simulink model "generic"  (R2021a)
settings: Solver=ode8  StartTime=0.0  StopTime=inf  FixedStep=0.001  RelTol=1e-3  EnableMultiTasking=on
StartFcn:
  | addpath('C:\Stud\Mgr_work\casadi-windows-matlabR2016a-v3.5.5')
  | import casadi.*
libraries: CarMaker4SL x35, simulink x1
(part 3 of 3)

== system generic/CarMaker/VehicleControl/CreateBus VhclCtrl/Environmental Envelope Protection/MPC/for ruts/Subsystem3 ==
  In1 : Inport
  Bus Selector{1..10} (10 alike) : BusSelector  OutputSignals=x,y,z
  Mux : Mux  Inputs=10
  Mux1 : Mux  Inputs=10
  Selector1 : Selector  InputPortWidth=200  IndexOptions=Index vector (dialog)  Indices=1  OutputSizes=1
  Selector10 : Selector  InputPortWidth=200  IndexOptions=Index vector (dialog)  Indices=10  OutputSizes=1
  Selector2 : Selector  InputPortWidth=200  IndexOptions=Index vector (dialog)  Indices=2  OutputSizes=1
  Selector3 : Selector  InputPortWidth=200  IndexOptions=Index vector (dialog)  Indices=3  OutputSizes=1
  Selector4 : Selector  InputPortWidth=200  IndexOptions=Index vector (dialog)  Indices=4  OutputSizes=1
  Selector5 : Selector  InputPortWidth=200  IndexOptions=Index vector (dialog)  Indices=5  OutputSizes=1
  Selector6 : Selector  InputPortWidth=200  IndexOptions=Index vector (dialog)  Indices=6  OutputSizes=1
  Selector7 : Selector  InputPortWidth=200  IndexOptions=Index vector (dialog)  Indices=7  OutputSizes=1
  Selector8 : Selector  InputPortWidth=200  IndexOptions=Index vector (dialog)  Indices=8  OutputSizes=1
  Selector9 : Selector  InputPortWidth=200  IndexOptions=Index vector (dialog)  Indices=9  OutputSizes=1
  x : Outport
  y : Outport  Port=2
  wires:
  Bus Selector1/1 -> Mux/1  "<x>"
  Bus Selector2/2 -> Mux1/2  "<y>"
  In1/1 -> Selector2/1, Selector10/1, Selector9/1, Selector8/1, Selector7/1, Selector6/1, Selector5/1, Selector4/1, Selector3/1, Selector1/1
  Bus Selector2/1 -> Mux/2  "<x>"
  Selector2/1 -> Bus Selector2/1
  Selector1/1 -> Bus Selector1/1
  Bus Selector1/2 -> Mux1/1  "<y>"
  Bus Selector3/1 -> Mux/3  "<x>"
  Bus Selector3/2 -> Mux1/3  "<y>"
  Selector3/1 -> Bus Selector3/1
  Bus Selector4/1 -> Mux/4  "<x>"
  Bus Selector4/2 -> Mux1/4  "<y>"
  Selector4/1 -> Bus Selector4/1
  Bus Selector5/1 -> Mux/5  "<x>"
  Bus Selector5/2 -> Mux1/5  "<y>"
  Selector5/1 -> Bus Selector5/1
  Bus Selector6/1 -> Mux/6  "<x>"
  Bus Selector6/2 -> Mux1/6  "<y>"
  Selector6/1 -> Bus Selector6/1
  Bus Selector7/1 -> Mux/7  "<x>"
  Bus Selector7/2 -> Mux1/7  "<y>"
  Selector7/1 -> Bus Selector7/1
  Bus Selector8/1 -> Mux/8  "<x>"
  Bus Selector8/2 -> Mux1/8  "<y>"
  Selector8/1 -> Bus Selector8/1
  Bus Selector9/1 -> Mux/9  "<x>"
  Bus Selector9/2 -> Mux1/9  "<y>"
  Selector9/1 -> Bus Selector9/1
  Bus Selector10/1 -> Mux/10  "<x>"
  Bus Selector10/2 -> Mux1/10  "<y>"
  Selector10/1 -> Bus Selector10/1
  Mux1/1 -> y/1
  Mux/1 -> x/1

== system generic/CarMaker/VehicleControl/CreateBus VhclCtrl/Environmental Envelope Protection/MPC/for ruts/Subsystem4 ==
  In1 : Inport
  Bus Selector{1..10} (10 alike) : BusSelector  OutputSignals=x,y,z
  Mux : Mux  Inputs=10
  Mux1 : Mux  Inputs=10
  Selector1 : Selector  InputPortWidth=200  IndexOptions=Index vector (dialog)  Indices=1  OutputSizes=1
  Selector10 : Selector  InputPortWidth=200  IndexOptions=Index vector (dialog)  Indices=10  OutputSizes=1
  Selector2 : Selector  InputPortWidth=200  IndexOptions=Index vector (dialog)  Indices=2  OutputSizes=1
  Selector3 : Selector  InputPortWidth=200  IndexOptions=Index vector (dialog)  Indices=3  OutputSizes=1
  Selector4 : Selector  InputPortWidth=200  IndexOptions=Index vector (dialog)  Indices=4  OutputSizes=1
  Selector5 : Selector  InputPortWidth=200  IndexOptions=Index vector (dialog)  Indices=5  OutputSizes=1
  Selector6 : Selector  InputPortWidth=200  IndexOptions=Index vector (dialog)  Indices=6  OutputSizes=1
  Selector7 : Selector  InputPortWidth=200  IndexOptions=Index vector (dialog)  Indices=7  OutputSizes=1
  Selector8 : Selector  InputPortWidth=200  IndexOptions=Index vector (dialog)  Indices=8  OutputSizes=1
  Selector9 : Selector  InputPortWidth=200  IndexOptions=Index vector (dialog)  Indices=9  OutputSizes=1
  x : Outport
  y : Outport  Port=2
  wires:
  Bus Selector1/1 -> Mux/1  "<x>"
  Bus Selector2/2 -> Mux1/2  "<y>"
  In1/1 -> Selector2/1, Selector10/1, Selector9/1, Selector8/1, Selector7/1, Selector6/1, Selector5/1, Selector4/1, Selector3/1, Selector1/1
  Bus Selector2/1 -> Mux/2  "<x>"
  Selector2/1 -> Bus Selector2/1
  Selector1/1 -> Bus Selector1/1
  Bus Selector1/2 -> Mux1/1  "<y>"
  Bus Selector3/1 -> Mux/3  "<x>"
  Bus Selector3/2 -> Mux1/3  "<y>"
  Selector3/1 -> Bus Selector3/1
  Bus Selector4/1 -> Mux/4  "<x>"
  Bus Selector4/2 -> Mux1/4  "<y>"
  Selector4/1 -> Bus Selector4/1
  Bus Selector5/1 -> Mux/5  "<x>"
  Bus Selector5/2 -> Mux1/5  "<y>"
  Selector5/1 -> Bus Selector5/1
  Bus Selector6/1 -> Mux/6  "<x>"
  Bus Selector6/2 -> Mux1/6  "<y>"
  Selector6/1 -> Bus Selector6/1
  Bus Selector7/1 -> Mux/7  "<x>"
  Bus Selector7/2 -> Mux1/7  "<y>"
  Selector7/1 -> Bus Selector7/1
  Bus Selector8/1 -> Mux/8  "<x>"
  Bus Selector8/2 -> Mux1/8  "<y>"
  Selector8/1 -> Bus Selector8/1
  Bus Selector9/1 -> Mux/9  "<x>"
  Bus Selector9/2 -> Mux1/9  "<y>"
  Selector9/1 -> Bus Selector9/1
  Bus Selector10/1 -> Mux/10  "<x>"
  Bus Selector10/2 -> Mux1/10  "<y>"
  Selector10/1 -> Bus Selector10/1
  Mux1/1 -> y/1
  Mux/1 -> x/1

== system generic/CarMaker/VehicleControl/CreateBus VhclCtrl/Environmental Envelope Protection/MPC/for ruts/Subsystem5 ==
  In1 : Inport
  Bus Selector{1..10} (10 alike) : BusSelector  OutputSignals=x,y,z
  Mux : Mux  Inputs=10
  Mux1 : Mux  Inputs=10
  Selector1 : Selector  InputPortWidth=200  IndexOptions=Index vector (dialog)  Indices=1  OutputSizes=1
  Selector10 : Selector  InputPortWidth=200  IndexOptions=Index vector (dialog)  Indices=10  OutputSizes=1
  Selector2 : Selector  InputPortWidth=200  IndexOptions=Index vector (dialog)  Indices=2  OutputSizes=1
  Selector3 : Selector  InputPortWidth=200  IndexOptions=Index vector (dialog)  Indices=3  OutputSizes=1
  Selector4 : Selector  InputPortWidth=200  IndexOptions=Index vector (dialog)  Indices=4  OutputSizes=1
  Selector5 : Selector  InputPortWidth=200  IndexOptions=Index vector (dialog)  Indices=5  OutputSizes=1
  Selector6 : Selector  InputPortWidth=200  IndexOptions=Index vector (dialog)  Indices=6  OutputSizes=1
  Selector7 : Selector  InputPortWidth=200  IndexOptions=Index vector (dialog)  Indices=7  OutputSizes=1
  Selector8 : Selector  InputPortWidth=200  IndexOptions=Index vector (dialog)  Indices=8  OutputSizes=1
  Selector9 : Selector  InputPortWidth=200  IndexOptions=Index vector (dialog)  Indices=9  OutputSizes=1
  x : Outport
  y : Outport  Port=2
  wires:
  Bus Selector1/1 -> Mux/1  "<x>"
  Bus Selector2/2 -> Mux1/2  "<y>"
  In1/1 -> Selector2/1, Selector10/1, Selector9/1, Selector8/1, Selector7/1, Selector6/1, Selector5/1, Selector4/1, Selector3/1, Selector1/1
  Bus Selector2/1 -> Mux/2  "<x>"
  Selector2/1 -> Bus Selector2/1
  Selector1/1 -> Bus Selector1/1
  Bus Selector1/2 -> Mux1/1  "<y>"
  Bus Selector3/1 -> Mux/3  "<x>"
  Bus Selector3/2 -> Mux1/3  "<y>"
  Selector3/1 -> Bus Selector3/1
  Bus Selector4/1 -> Mux/4  "<x>"
  Bus Selector4/2 -> Mux1/4  "<y>"
  Selector4/1 -> Bus Selector4/1
  Bus Selector5/1 -> Mux/5  "<x>"
  Bus Selector5/2 -> Mux1/5  "<y>"
  Selector5/1 -> Bus Selector5/1
  Bus Selector6/1 -> Mux/6  "<x>"
  Bus Selector6/2 -> Mux1/6  "<y>"
  Selector6/1 -> Bus Selector6/1
  Bus Selector7/1 -> Mux/7  "<x>"
  Bus Selector7/2 -> Mux1/7  "<y>"
  Selector7/1 -> Bus Selector7/1
  Bus Selector8/1 -> Mux/8  "<x>"
  Bus Selector8/2 -> Mux1/8  "<y>"
  Selector8/1 -> Bus Selector8/1
  Bus Selector9/1 -> Mux/9  "<x>"
  Bus Selector9/2 -> Mux1/9  "<y>"
  Selector9/1 -> Bus Selector9/1
  Bus Selector10/1 -> Mux/10  "<x>"
  Bus Selector10/2 -> Mux1/10  "<y>"
  Selector10/1 -> Bus Selector10/1
  Mux1/1 -> y/1
  Mux/1 -> x/1

== system generic/CarMaker/VehicleControl/CreateBus VhclCtrl/Environmental Envelope Protection/MPC/for ruts/Subsystem6 ==
  In1 : Inport
  Bus Selector{1..10} (10 alike) : BusSelector  OutputSignals=x,y,z
  Mux : Mux  Inputs=10
  Mux1 : Mux  Inputs=10
  Selector1 : Selector  InputPortWidth=200  IndexOptions=Index vector (dialog)  Indices=1  OutputSizes=1
  Selector10 : Selector  InputPortWidth=200  IndexOptions=Index vector (dialog)  Indices=10  OutputSizes=1
  Selector2 : Selector  InputPortWidth=200  IndexOptions=Index vector (dialog)  Indices=2  OutputSizes=1
  Selector3 : Selector  InputPortWidth=200  IndexOptions=Index vector (dialog)  Indices=3  OutputSizes=1
  Selector4 : Selector  InputPortWidth=200  IndexOptions=Index vector (dialog)  Indices=4  OutputSizes=1
  Selector5 : Selector  InputPortWidth=200  IndexOptions=Index vector (dialog)  Indices=5  OutputSizes=1
  Selector6 : Selector  InputPortWidth=200  IndexOptions=Index vector (dialog)  Indices=6  OutputSizes=1
  Selector7 : Selector  InputPortWidth=200  IndexOptions=Index vector (dialog)  Indices=7  OutputSizes=1
  Selector8 : Selector  InputPortWidth=200  IndexOptions=Index vector (dialog)  Indices=8  OutputSizes=1
  Selector9 : Selector  InputPortWidth=200  IndexOptions=Index vector (dialog)  Indices=9  OutputSizes=1
  x : Outport
  y : Outport  Port=2
  wires:
  Bus Selector1/1 -> Mux/1  "<x>"
  Bus Selector2/2 -> Mux1/2  "<y>"
  In1/1 -> Selector2/1, Selector10/1, Selector9/1, Selector8/1, Selector7/1, Selector6/1, Selector5/1, Selector4/1, Selector3/1, Selector1/1
  Bus Selector2/1 -> Mux/2  "<x>"
  Selector2/1 -> Bus Selector2/1
  Selector1/1 -> Bus Selector1/1
  Bus Selector1/2 -> Mux1/1  "<y>"
  Bus Selector3/1 -> Mux/3  "<x>"
  Bus Selector3/2 -> Mux1/3  "<y>"
  Selector3/1 -> Bus Selector3/1
  Bus Selector4/1 -> Mux/4  "<x>"
  Bus Selector4/2 -> Mux1/4  "<y>"
  Selector4/1 -> Bus Selector4/1
  Bus Selector5/1 -> Mux/5  "<x>"
  Bus Selector5/2 -> Mux1/5  "<y>"
  Selector5/1 -> Bus Selector5/1
  Bus Selector6/1 -> Mux/6  "<x>"
  Bus Selector6/2 -> Mux1/6  "<y>"
  Selector6/1 -> Bus Selector6/1
  Bus Selector7/1 -> Mux/7  "<x>"
  Bus Selector7/2 -> Mux1/7  "<y>"
  Selector7/1 -> Bus Selector7/1
  Bus Selector8/1 -> Mux/8  "<x>"
  Bus Selector8/2 -> Mux1/8  "<y>"
  Selector8/1 -> Bus Selector8/1
  Bus Selector9/1 -> Mux/9  "<x>"
  Bus Selector9/2 -> Mux1/9  "<y>"
  Selector9/1 -> Bus Selector9/1
  Bus Selector10/1 -> Mux/10  "<x>"
  Bus Selector10/2 -> Mux1/10  "<y>"
  Selector10/1 -> Bus Selector10/1
  Mux1/1 -> y/1
  Mux/1 -> x/1

== system generic/CarMaker/VehicleControl/CreateBus VhclCtrl/Environmental Envelope Protection/MPC/for ruts/Subsystem7 ==
  In1 : Inport
  Bus Selector{1..10} (10 alike) : BusSelector  OutputSignals=x,y,z
  Mux : Mux  Inputs=10
  Mux1 : Mux  Inputs=10
  Selector1 : Selector  InputPortWidth=200  IndexOptions=Index vector (dialog)  Indices=1  OutputSizes=1
  Selector10 : Selector  InputPortWidth=200  IndexOptions=Index vector (dialog)  Indices=10  OutputSizes=1
  Selector2 : Selector  InputPortWidth=200  IndexOptions=Index vector (dialog)  Indices=2  OutputSizes=1
  Selector3 : Selector  InputPortWidth=200  IndexOptions=Index vector (dialog)  Indices=3  OutputSizes=1
  Selector4 : Selector  InputPortWidth=200  IndexOptions=Index vector (dialog)  Indices=4  OutputSizes=1
  Selector5 : Selector  InputPortWidth=200  IndexOptions=Index vector (dialog)  Indices=5  OutputSizes=1
  Selector6 : Selector  InputPortWidth=200  IndexOptions=Index vector (dialog)  Indices=6  OutputSizes=1
  Selector7 : Selector  InputPortWidth=200  IndexOptions=Index vector (dialog)  Indices=7  OutputSizes=1
  Selector8 : Selector  InputPortWidth=200  IndexOptions=Index vector (dialog)  Indices=8  OutputSizes=1
  Selector9 : Selector  InputPortWidth=200  IndexOptions=Index vector (dialog)  Indices=9  OutputSizes=1
  x : Outport
  y : Outport  Port=2
  wires:
  Bus Selector1/1 -> Mux/1  "<x>"
  Bus Selector2/2 -> Mux1/2  "<y>"
  In1/1 -> Selector2/1, Selector10/1, Selector9/1, Selector8/1, Selector7/1, Selector6/1, Selector5/1, Selector4/1, Selector3/1, Selector1/1
  Bus Selector2/1 -> Mux/2  "<x>"
  Selector2/1 -> Bus Selector2/1
  Selector1/1 -> Bus Selector1/1
  Bus Selector1/2 -> Mux1/1  "<y>"
  Bus Selector3/1 -> Mux/3  "<x>"
  Bus Selector3/2 -> Mux1/3  "<y>"
  Selector3/1 -> Bus Selector3/1
  Bus Selector4/1 -> Mux/4  "<x>"
  Bus Selector4/2 -> Mux1/4  "<y>"
  Selector4/1 -> Bus Selector4/1
  Bus Selector5/1 -> Mux/5  "<x>"
  Bus Selector5/2 -> Mux1/5  "<y>"
  Selector5/1 -> Bus Selector5/1
  Bus Selector6/1 -> Mux/6  "<x>"
  Bus Selector6/2 -> Mux1/6  "<y>"
  Selector6/1 -> Bus Selector6/1
  Bus Selector7/1 -> Mux/7  "<x>"
  Bus Selector7/2 -> Mux1/7  "<y>"
  Selector7/1 -> Bus Selector7/1
  Bus Selector8/1 -> Mux/8  "<x>"
  Bus Selector8/2 -> Mux1/8  "<y>"
  Selector8/1 -> Bus Selector8/1
  Bus Selector9/1 -> Mux/9  "<x>"
  Bus Selector9/2 -> Mux1/9  "<y>"
  Selector9/1 -> Bus Selector9/1
  Bus Selector10/1 -> Mux/10  "<x>"
  Bus Selector10/2 -> Mux1/10  "<y>"
  Selector10/1 -> Bus Selector10/1
  Mux1/1 -> y/1
  Mux/1 -> x/1

== system generic/CarMaker/VehicleControl/CreateBus VhclCtrl/Environmental Envelope Protection/MPC/for ruts/Subsystem8 ==
  In1 : Inport
  Bus Selector{1..10} (10 alike) : BusSelector  OutputSignals=x,y,z
  Mux : Mux  Inputs=10
  Mux1 : Mux  Inputs=10
  Selector1 : Selector  InputPortWidth=200  IndexOptions=Index vector (dialog)  Indices=1  OutputSizes=1
  Selector10 : Selector  InputPortWidth=200  IndexOptions=Index vector (dialog)  Indices=10  OutputSizes=1
  Selector2 : Selector  InputPortWidth=200  IndexOptions=Index vector (dialog)  Indices=2  OutputSizes=1
  Selector3 : Selector  InputPortWidth=200  IndexOptions=Index vector (dialog)  Indices=3  OutputSizes=1
  Selector4 : Selector  InputPortWidth=200  IndexOptions=Index vector (dialog)  Indices=4  OutputSizes=1
  Selector5 : Selector  InputPortWidth=200  IndexOptions=Index vector (dialog)  Indices=5  OutputSizes=1
  Selector6 : Selector  InputPortWidth=200  IndexOptions=Index vector (dialog)  Indices=6  OutputSizes=1
  Selector7 : Selector  InputPortWidth=200  IndexOptions=Index vector (dialog)  Indices=7  OutputSizes=1
  Selector8 : Selector  InputPortWidth=200  IndexOptions=Index vector (dialog)  Indices=8  OutputSizes=1
  Selector9 : Selector  InputPortWidth=200  IndexOptions=Index vector (dialog)  Indices=9  OutputSizes=1
  x : Outport
  y : Outport  Port=2
  wires:
  Bus Selector1/1 -> Mux/1  "<x>"
  Bus Selector2/2 -> Mux1/2  "<y>"
  In1/1 -> Selector2/1, Selector10/1, Selector9/1, Selector8/1, Selector7/1, Selector6/1, Selector5/1, Selector4/1, Selector3/1, Selector1/1
  Bus Selector2/1 -> Mux/2  "<x>"
  Selector2/1 -> Bus Selector2/1
  Selector1/1 -> Bus Selector1/1
  Bus Selector1/2 -> Mux1/1  "<y>"
  Bus Selector3/1 -> Mux/3  "<x>"
  Bus Selector3/2 -> Mux1/3  "<y>"
  Selector3/1 -> Bus Selector3/1
  Bus Selector4/1 -> Mux/4  "<x>"
  Bus Selector4/2 -> Mux1/4  "<y>"
  Selector4/1 -> Bus Selector4/1
  Bus Selector5/1 -> Mux/5  "<x>"
  Bus Selector5/2 -> Mux1/5  "<y>"
  Selector5/1 -> Bus Selector5/1
  Bus Selector6/1 -> Mux/6  "<x>"
  Bus Selector6/2 -> Mux1/6  "<y>"
  Selector6/1 -> Bus Selector6/1
  Bus Selector7/1 -> Mux/7  "<x>"
  Bus Selector7/2 -> Mux1/7  "<y>"
  Selector7/1 -> Bus Selector7/1
  Bus Selector8/1 -> Mux/8  "<x>"
  Bus Selector8/2 -> Mux1/8  "<y>"
  Selector8/1 -> Bus Selector8/1
  Bus Selector9/1 -> Mux/9  "<x>"
  Bus Selector9/2 -> Mux1/9  "<y>"
  Selector9/1 -> Bus Selector9/1
  Bus Selector10/1 -> Mux/10  "<x>"
  Bus Selector10/2 -> Mux1/10  "<y>"
  Selector10/1 -> Bus Selector10/1
  Mux1/1 -> y/1
  Mux/1 -> x/1

== system generic/CarMaker/VehicleControl/CreateBus VhclCtrl/Environmental Envelope Protection/MPC/for ruts/Subsystem9 ==
  In1 : Inport
  Bus Selector{1..10} (10 alike) : BusSelector  OutputSignals=x,y,z
  Mux : Mux  Inputs=10
  Mux1 : Mux  Inputs=10
  Selector1 : Selector  InputPortWidth=200  IndexOptions=Index vector (dialog)  Indices=1  OutputSizes=1
  Selector10 : Selector  InputPortWidth=200  IndexOptions=Index vector (dialog)  Indices=10  OutputSizes=1
  Selector2 : Selector  InputPortWidth=200  IndexOptions=Index vector (dialog)  Indices=2  OutputSizes=1
  Selector3 : Selector  InputPortWidth=200  IndexOptions=Index vector (dialog)  Indices=3  OutputSizes=1
  Selector4 : Selector  InputPortWidth=200  IndexOptions=Index vector (dialog)  Indices=4  OutputSizes=1
  Selector5 : Selector  InputPortWidth=200  IndexOptions=Index vector (dialog)  Indices=5  OutputSizes=1
  Selector6 : Selector  InputPortWidth=200  IndexOptions=Index vector (dialog)  Indices=6  OutputSizes=1
  Selector7 : Selector  InputPortWidth=200  IndexOptions=Index vector (dialog)  Indices=7  OutputSizes=1
  Selector8 : Selector  InputPortWidth=200  IndexOptions=Index vector (dialog)  Indices=8  OutputSizes=1
  Selector9 : Selector  InputPortWidth=200  IndexOptions=Index vector (dialog)  Indices=9  OutputSizes=1
  x : Outport
  y : Outport  Port=2
  wires:
  Bus Selector1/1 -> Mux/1  "<x>"
  Bus Selector2/2 -> Mux1/2  "<y>"
  In1/1 -> Selector2/1, Selector10/1, Selector9/1, Selector8/1, Selector7/1, Selector6/1, Selector5/1, Selector4/1, Selector3/1, Selector1/1
  Bus Selector2/1 -> Mux/2  "<x>"
  Selector2/1 -> Bus Selector2/1
  Selector1/1 -> Bus Selector1/1
  Bus Selector1/2 -> Mux1/1  "<y>"
  Bus Selector3/1 -> Mux/3  "<x>"
  Bus Selector3/2 -> Mux1/3  "<y>"
  Selector3/1 -> Bus Selector3/1
  Bus Selector4/1 -> Mux/4  "<x>"
  Bus Selector4/2 -> Mux1/4  "<y>"
  Selector4/1 -> Bus Selector4/1
  Bus Selector5/1 -> Mux/5  "<x>"
  Bus Selector5/2 -> Mux1/5  "<y>"
  Selector5/1 -> Bus Selector5/1
  Bus Selector6/1 -> Mux/6  "<x>"
  Bus Selector6/2 -> Mux1/6  "<y>"
  Selector6/1 -> Bus Selector6/1
  Bus Selector7/1 -> Mux/7  "<x>"
  Bus Selector7/2 -> Mux1/7  "<y>"
  Selector7/1 -> Bus Selector7/1
  Bus Selector8/1 -> Mux/8  "<x>"
  Bus Selector8/2 -> Mux1/8  "<y>"
  Selector8/1 -> Bus Selector8/1
  Bus Selector9/1 -> Mux/9  "<x>"
  Bus Selector9/2 -> Mux1/9  "<y>"
  Selector9/1 -> Bus Selector9/1
  Bus Selector10/1 -> Mux/10  "<x>"
  Bus Selector10/2 -> Mux1/10  "<y>"
  Selector10/1 -> Bus Selector10/1
  Mux1/1 -> y/1
  Mux/1 -> x/1

== matlab function generic/CarMaker/VehicleControl/CreateBus VhclCtrl/Environmental Envelope Protection/MPC/for ruts/MATLAB Function1 ==
  data: points_x output; line_id input; ids input; points_y output; X input; Y input
function [points_x, points_y]  = line_id_points(line_id, ids, X, Y)

% line_id = 8; %main left line
% id_main_left_left = 18;
% id_main_left_right = 17;
% id_main_right_left = 15;
% id_main_right_right = 16;
% id_main_right = 19;

% shifts according to cg from sensor's placement approx
shifts = [0.75, 0.8;
          0.75, 0.8;
          0.75, 1.4;
          0.75, 1.4;
          0.75, 0;
          0.75, 0;
          0.75, -0.8;
          0.75, -0.8;
          0.75, -1.4;
          0.75, -1.4];

points_x = zeros(10,1);
points_y = zeros(10,1);

row_number = find(ids == line_id, 1, 'first');

if(~isempty(row_number))
    points_x(:) = X(:,row_number) + ones(10,1)*shifts(row_number, 1);
    points_y(:) = Y(:,row_number) + ones(10,1)*shifts(row_number, 2);
end

== matlab function generic/CarMaker/VehicleControl/CreateBus VhclCtrl/Environmental Envelope Protection/MPC/for ruts/MATLAB Function2 ==
  data: points_x output; line_id input; ids input; points_y output; X input; Y input
function [points_x, points_y]  = line_id_points(line_id, ids, X, Y)

% line_id = 8; %main left line
% id_main_left_left = 18;
% id_main_left_right = 17;
% id_main_right_left = 15;
% id_main_right_right = 16;
% id_main_right = 19;

% shifts according to cg from sensor's placement approx
shifts = [0.75, 0.8;
          0.75, 0.8;
          0.75, 1.4;
          0.75, 1.4;
          0.75, 0;
          0.75, 0;
          0.75, -0.8;
          0.75, -0.8;
          0.75, -1.4;
          0.75, -1.4];

points_x = zeros(10,1);
points_y = zeros(10,1);

row_number = find(ids == line_id, 1, 'first');

if(~isempty(row_number))
    points_x(:) = X(:,row_number) + ones(10,1)*shifts(row_number, 1);
    points_y(:) = Y(:,row_number) + ones(10,1)*shifts(row_number, 2);
end

== matlab function generic/CarMaker/VehicleControl/CreateBus VhclCtrl/Environmental Envelope Protection/MPC/for ruts/MATLAB Function3 ==
  data: points_x output; line_id input; ids input; points_y output; X input; Y input
function [points_x, points_y]  = line_id_points(line_id, ids, X, Y)

% line_id = 8; %main left line
% id_main_left_left = 18;
% id_main_left_right = 17;
% id_main_right_left = 15;
% id_main_right_right = 16;
% id_main_right = 19;

% shifts according to cg from sensor's placement approx
shifts = [0.75, 0.8;
          0.75, 0.8;
          0.75, 1.4;
          0.75, 1.4;
          0.75, 0;
          0.75, 0;
          0.75, -0.8;
          0.75, -0.8;
          0.75, -1.4;
          0.75, -1.4];

points_x = zeros(10,1);
points_y = zeros(10,1);

row_number = find(ids == line_id, 1, 'first');

if(~isempty(row_number))
    points_x(:) = X(:,row_number) + ones(10,1)*shifts(row_number, 1);
    points_y(:) = Y(:,row_number) + ones(10,1)*shifts(row_number, 2);
end

== matlab function generic/CarMaker/VehicleControl/CreateBus VhclCtrl/Environmental Envelope Protection/MPC/for ruts/MATLAB Function4 ==
  data: points_x output; line_id input; ids input; points_y output; X input; Y input
function [points_x, points_y]  = line_id_points(line_id, ids, X, Y)

% line_id = 8; %main left line
% id_main_left_left = 18;
% id_main_left_right = 17;
% id_main_right_left = 15;
% id_main_right_right = 16;
% id_main_right = 19;

% shifts according to cg from sensor's placement approx
shifts = [0.75, 0.8;
          0.75, 0.8;
          0.75, 1.4;
          0.75, 1.4;
          0.75, 0;
          0.75, 0;
          0.75, -0.8;
          0.75, -0.8;
          0.75, -1.4;
          0.75, -1.4];

points_x = zeros(10,1);
points_y = zeros(10,1);

row_number = find(ids == line_id, 1, 'first');

if(~isempty(row_number))
    points_x(:) = X(:,row_number) + ones(10,1)*shifts(row_number, 1);
    points_y(:) = Y(:,row_number) + ones(10,1)*shifts(row_number, 2);
end

== matlab function generic/CarMaker/VehicleControl/CreateBus VhclCtrl/Environmental Envelope Protection/MPC/for ruts/MATLAB Function5 ==
  data: points_x output; line_id input; ids input; points_y output; X input; Y input
function [points_x, points_y]  = line_id_points(line_id, ids, X, Y)

% line_id = 8; %main left line
% id_main_left_left = 18;
% id_main_left_right = 17;
% id_main_right_left = 15;
% id_main_right_right = 16;
% id_main_right = 19;

% shifts according to cg from sensor's placement approx
shifts = [0.75, 0.8;
          0.75, 0.8;
          0.75, 1.4;
          0.75, 1.4;
          0.75, 0;
          0.75, 0;
          0.75, -0.8;
          0.75, -0.8;
          0.75, -1.4;
          0.75, -1.4];

points_x = zeros(10,1);
points_y = zeros(10,1);

row_number = find(ids == line_id, 1, 'first');

if(~isempty(row_number))
    points_x(:) = X(:,row_number) + ones(10,1)*shifts(row_number, 1);
    points_y(:) = Y(:,row_number) + ones(10,1)*shifts(row_number, 2);
end

== matlab function generic/CarMaker/VehicleControl/CreateBus VhclCtrl/Environmental Envelope Protection/MPC/SIgn detection for priority test/MATLAB Function ==
  data: point_x output; sing_id input; ids input; point_y output; X input; Y input
function [point_x, point_y]  = line_id_points(sing_id, ids, X, Y)

% child 13
% caution 11

point_x = 0;
point_y = 0;

row_number = find(ids == sing_id, 1, 'first');


if(~isempty(row_number))
    point_x = X(row_number(1));
    point_y = Y(row_number(1));
end

== matlab function generic/CarMaker/VehicleControl/CreateBus VhclCtrl/Environmental Envelope Protection/MPC/SIgn detection for priority test/MATLAB Function1 ==
  data: point_x output; sing_id input; ids input; point_y output; X input; Y input
function [point_x, point_y]  = line_id_points(sing_id, ids, X, Y)

% child 13
% caution 11

point_x = 0;
point_y = 0;

row_number = find(ids == sing_id, 1, 'first');


if(~isempty(row_number))
    point_x = X(row_number(1));
    point_y = Y(row_number(1));
end

== matlab function generic/CarMaker/VehicleControl/CreateBus VhclCtrl/Environmental Envelope Protection/Control switcher with memory/MATLAB Function ==
  data: v input; control_on output; thr input
function control_on = fcn(v, thr)
if(v >= thr)
    control_on = 1;
else
    control_on = -1;
end

== matlab function generic/CarMaker/VehicleControl/CreateBus VhclCtrl/Environmental Envelope Protection/MATLAB Function ==
  data: t input; y output; t_ctrl_on input; override_off input; velocity_flag input
function y = fcn(t, t_ctrl_on, override_off, velocity_flag)
% sends -1 for control off, 1 for control on
if (override_off)
    y = -1;
else
    if(t < t_ctrl_on || velocity_flag ~= 1)
        y = -1;
    else
        y = 1;
    end 
end

== matlab function generic/CarMaker/VehicleControl/CreateBus VhclCtrl/Environmental Envelope Protection/start time selector ==
  data: u input; y output
function y = fcn(u)

switch u
   case 0
      y = 30;
   case 1
      y = 22;
   case 2
      y = 18;
   case 3
      y = 22;
   case 4
      y = 20;
   case 5
      y = 20;
   case 6
      y = 22;
   otherwise
      y = 0;
end

== matlab function generic/CarMaker/VehicleControl/CreateBus VhclCtrl/Environmental Envelope Protection/MPC/MPC LTI Strategy ==
  data: t input; input input; u output; params input; controller_on input; points_x_r input; points_x_l input; points_y_r input; points_y_l input; obstacle_flag input; ds_x input; ds_y input; SignDetections input; TestCase input; LineDetections input
function u = fcn(t, input, params, controller_on, points_x_r, points_x_l, points_y_r, points_y_l, obstacle_flag, ds_x, ds_y, SignDetections, TestCase, LineDetections)

coder.extrinsic('main_mpc')
coder.extrinsic('mpc_for_sign_priority')
coder.extrinsic('main_mpc_undrivable_obstacle')
coder.extrinsic('mpc_for_rutroad')
u = 0;

if TestCase == 0 || TestCase == 1 || TestCase == 2

    u = main_mpc(t, input, params, controller_on, points_x_r, points_x_l, points_y_r, points_y_l, obstacle_flag, ds_x, ds_y);

end

if TestCase == 3

    u = main_mpc_undrivable_obstacle(t, input, params, controller_on, points_x_r, points_x_l, points_y_r, points_y_l, obstacle_flag, ds_x, ds_y);

end

if TestCase == 4 || TestCase == 5

    u = mpc_for_sign_priority(t, input, params, controller_on, points_x_r, points_x_l, points_y_r, points_y_l, obstacle_flag, ds_x, ds_y, SignDetections);

end

if TestCase == 6

    u = mpc_for_rutroad(t, input, params, controller_on, LineDetections);
end

== matlab function generic/CarMaker/VehicleControl/CreateBus VhclCtrl/Environmental Envelope Protection/MPC/for ruts/MATLAB Function ==
  data: points_x output; line_id input; ids input; points_y output; X input; Y input
function [points_x, points_y]  = line_id_points(line_id, ids, X, Y)

% line_id = 8; %main left line
% id_main_left_left = 18;
% id_main_left_right = 17;
% id_main_right_left = 15;
% id_main_right_right = 16;
% id_main_right = 19;

% shifts according to cg from sensor's placement approx
shifts = [0.75, 0.8;
          0.75, 0.8;
          0.75, 1.4;
          0.75, 1.4;
          0.75, 0;
          0.75, 0;
          0.75, -0.8;
          0.75, -0.8;
          0.75, -1.4;
          0.75, -1.4];

points_x = zeros(10,1);
points_y = zeros(10,1);

row_number = find(ids == line_id, 1, 'first');

if(~isempty(row_number))
    points_x(:) = X(:,row_number) + ones(10,1)*shifts(row_number, 1);
    points_y(:) = Y(:,row_number) + ones(10,1)*shifts(row_number, 2);
end
